simulink model "PowerTrainModeling"  (R2016a)
settings: Solver=ode3  StartTime=0.0  StopTime=1220  FixedStep=0.1  RelTol=1e-3
libraries: simulink x6
(part 3 of 3)

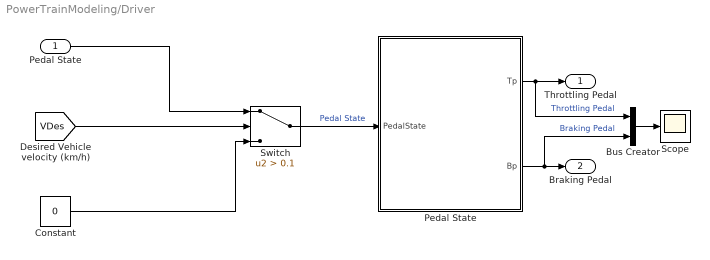
== system PowerTrainModeling/Driver ==
  "Pedal State " : Inport
  Bus Creator : BusCreator  Inputs=2
  Constant : Constant  Value=0
  Pedal State : MATLAB Function  TreatAsAtomicUnit=on
  Scope : Scope
  Switch : Switch  Criteria=u2 > Threshold  Threshold=0.1
  Throttling Pedal : Outport
  Braking Pedal : Outport  Port=2
  wires:
  Pedal State/2(Bp) -> Bus Creator/2, Braking Pedal/1  "Braking Pedal"
  Switch/1 -> Pedal State/1(PedalState)  "Pedal State"
  Constant/1 -> Switch/3
  [VDes] -> Switch/2
  Pedal State/1(Tp) -> Bus Creator/1, Throttling Pedal/1  "Throttling Pedal"
  "Pedal State "/1 -> Switch/1
  Bus Creator/1 -> Scope/1

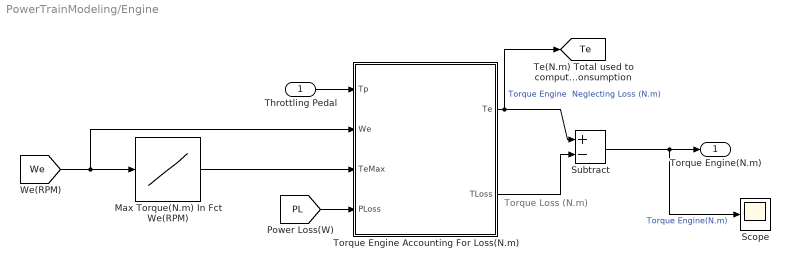
== system PowerTrainModeling/Engine  ==
  note: Torque Loss
      | (N.m)
  Throttling Pedal : Inport
  Max Torque(N.m) In Fct We(RPM) : Lookup_n-D  NumberOfTableDimensions=1  BreakpointsForDimension1=|  Table=|  RndMeth=Simplest  InputSameDT=on
      BreakpointsForDimension1=|
      | [500
      | 1000
      | 1500
      | 2000
      | 2500
      | 3000
      | 3500
      | 4000
      | 4500
      | 5000
      | 5500
      | 6000
      | ]
      Table=|
      | [112.32
      | 134.16
      | 146.64
      | 158.34
      | 165.36
      | 162.24
      | 159.12
      | 159.9
      | 165.36
      | 164.58
      | 160.68
      | 151.32
      | ]
  Scope : Scope
  Subtract : Sum  Inputs=+-
  Torque Engine Accounting For Loss(N.m) : MATLAB Function  TreatAsAtomicUnit=on
  Torque Engine(N.m) : Outport
  tag scope: Te=global
  wires:
  Max Torque(N.m) In Fct We(RPM)/1 -> Torque Engine Accounting For Loss(N.m)/3(TeMax)
  Torque Engine Accounting For Loss(N.m)/1(Te) -> [Te], Subtract/1  "Torque Engine  Neglecting Loss (N.m)"
  Subtract/1 -> Scope/1, Torque Engine(N.m)/1  "Torque Engine(N.m)"
  Throttling Pedal/1 -> Torque Engine Accounting For Loss(N.m)/1(Tp)
  [PL] -> Torque Engine Accounting For Loss(N.m)/4(PLoss)
  Torque Engine Accounting For Loss(N.m)/2(TLoss) -> Subtract/2
  [We] -> Torque Engine Accounting For Loss(N.m)/2(We), Max Torque(N.m) In Fct We(RPM)/1

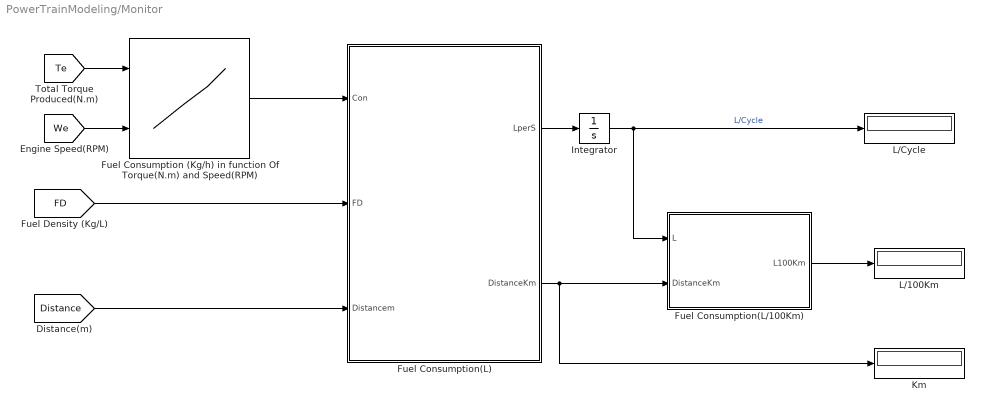
== system PowerTrainModeling/Monitor ==
  Fuel Consumption (Kg/h) in function Of Torque(N.m) and Speed(RPM) : Lookup_n-D  BreakpointsForDimension1=|  BreakpointsForDimension2=|  Table=|  RndMeth=Simplest  InputSameDT=on
      BreakpointsForDimension1=|
      | [15.6
      | 31.2
      | 46.8
      | 62.4
      | 78
      | 93.6
      | 109.2
      | 124.8
      | 140.4
      | 156
      | 171.6
      | ]
      Table=|
      | [0.50	1.00	1.50	1.94	2.28	2.56	2.68	3.41	3.97	5.59	6.79	7.41
      | 0.72	1.32	1.99	2.59	3.12	3.58	3.89	4.66	5.77	7.53	9.19	10.37
      | 0.91	1.65	2.54	3.28	3.93	4.58	4.94	6.22	7.75	9.26	11.35	12.70
      | 1.08	2.01	3.00	3.93	4.65	5.47	6.42	7.95	9.32	10.88	13.13	14.68
      | 1.25	2.32	3.44	4.50	5.44	6.44	7.92	9.23	10.78	12.50	14.72	16.41
      | 1.53	2.81	3.86	5.08	6.04	7.52	9.18	10.80	12.31	13.94	15.91	18.42
      | 1.73	3.23	4.37	5.60	7.00	8.52	10.37	12.02	13.99	16.20	18.79	20.50
      | 2.12	3.72	4.83	6.40	8.00	9.60	11.36	13.27	15.88	18.23	21.22	23.15
      | 2.12	4.23	5.56	7.30	9.00	10.80	12.78	15.46	18.05	20.80	23.58	25.72
      | 2.35	4.70	7.06	8.59	10.44	12.70	15.03	17.41	20.25	23.23	26.04	28.23
      | 2.59	5.18	7.76	10.35	12.94	15.53	18.11	20.70	23.29	25.88	28.46	31.05
      | ]
      BreakpointsForDimension2=|
      | [500	1000	1500	2000	2500	3000	3500	4000	4500	5000	5500	6000
      | ]
  Fuel Consumption(L) : MATLAB Function  TreatAsAtomicUnit=on
  Fuel Consumption(L/100Km) : MATLAB Function  TreatAsAtomicUnit=on
  Integrator : Integrator
  Km : Display
  L/100Km : Display
  L/Cycle : Display
  wires:
  [We] -> Fuel Consumption (Kg/h) in function Of Torque(N.m) and Speed(RPM)/2
  [Te] -> Fuel Consumption (Kg/h) in function Of Torque(N.m) and Speed(RPM)/1
  Fuel Consumption(L)/1(LperS) -> Integrator/1
  [FD] -> Fuel Consumption(L)/2(FD)
  Integrator/1 -> Fuel Consumption(L/100Km)/1(L), L/Cycle/1  "L/Cycle"
  Fuel Consumption(L)/2(DistanceKm) -> Km/1, Fuel Consumption(L/100Km)/2(DistanceKm)
  Fuel Consumption(L/100Km)/1(L100Km) -> L/100Km/1
  Fuel Consumption (Kg/h) in function Of Torque(N.m) and Speed(RPM)/1 -> Fuel Consumption(L)/1(Con)
  [Distance] -> Fuel Consumption(L)/3(Distancem)

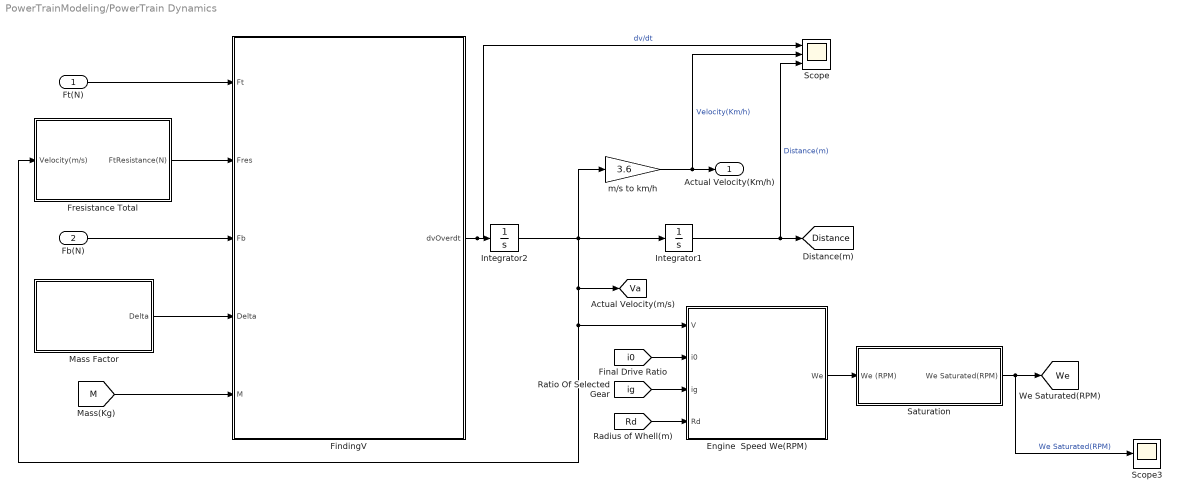
== system PowerTrainModeling/PowerTrain Dynamics  ==
  Ft(N) : Inport
  Fb(N) : Inport  Port=2
  Engine  Speed We(RPM) : MATLAB Function  TreatAsAtomicUnit=on
  FindingV : MATLAB Function  TreatAsAtomicUnit=on
  "Fresistance Total " : Subsystem
  Integrator1 : Integrator
  Integrator2 : Integrator
  Mass Factor : Subsystem
  Saturation : Subsystem
  Scope : Scope  NumInputPorts=3
  Scope3 : Scope
  m/s to km/h : Gain  Gain=3.6
  " Actual Velocity(Km/h)" : Outport
  tag scope: Distance=global, Va=global, We=global
  wires:
  "Fresistance Total "/1(FtResistance(N)) -> FindingV/2(Fres)
  Integrator1/1 -> Scope/3, [Distance]  "Distance(m)"
  FindingV/1(dvOverdt) -> Scope/1, Integrator2/1  "dv/dt"
  [M] -> FindingV/5(M)
  Ft(N)/1 -> FindingV/1(Ft)
  Mass Factor/1(Delta) -> FindingV/4(Delta)
  m/s to km/h/1 -> Scope/2, " Actual Velocity(Km/h)"/1  "Velocity(Km/h)"
  Fb(N)/1 -> FindingV/3(Fb)
  [ig] -> Engine  Speed We(RPM)/3(ig)
  [i0] -> Engine  Speed We(RPM)/2(i0)
  [Rd] -> Engine  Speed We(RPM)/4(Rd)
  Engine  Speed We(RPM)/1(We) -> Saturation/1(We (RPM))
  Saturation/1(We Saturated(RPM)) -> Scope3/1, [We]  "We Saturated(RPM)"
  Integrator2/1 -> m/s to km/h/1, Integrator1/1, "Fresistance Total "/1(Velocity(m/s)), Engine  Speed We(RPM)/1(V), [Va]

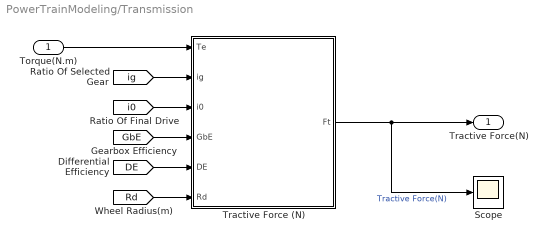
== system PowerTrainModeling/Transmission ==
  Torque(N.m) : Inport
  Scope : Scope
  Tractive Force (N) : MATLAB Function  TreatAsAtomicUnit=on
  Tractive Force(N) : Outport
  wires:
  [DE] -> Tractive Force (N)/5(DE)
  [i0] -> Tractive Force (N)/3(i0)
  [GbE] -> Tractive Force (N)/4(GbE)
  [Rd] -> Tractive Force (N)/6(Rd)
  [ig] -> Tractive Force (N)/2(ig)
  Torque(N.m)/1 -> Tractive Force (N)/1(Te)
  Tractive Force (N)/1(Ft) -> Scope/1, Tractive Force(N)/1  "Tractive Force(N)"

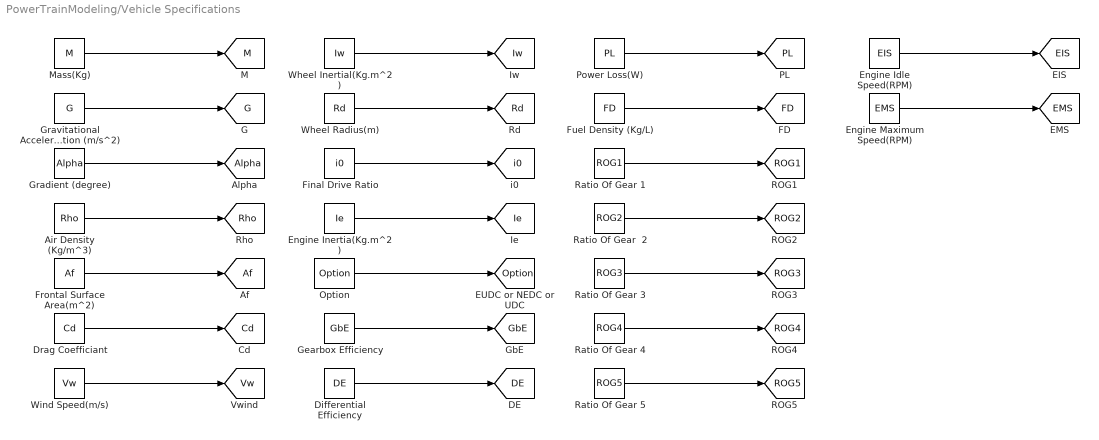
== system PowerTrainModeling/Vehicle Specifications ==
  Air Density (Kg/m^3) : Constant  Value=Rho
  Differential Efficiency : Constant  Value=DE
  Drag Coefficiant : Constant  Value=Cd
  Engine Idle Speed(RPM) : Constant  Value=EIS
  Engine Inertia(Kg.m^2) : Constant  Value=Ie
  Engine Maximum Speed(RPM) : Constant  Value=EMS
  Final Drive Ratio : Constant  Value=i0
  Frontal Surface Area(m^2) : Constant  Value=Af
  Fuel Density (Kg/L) : Constant  Value=FD
  Gearbox Efficiency : Constant  Value=GbE
  Gradient (degree) : Constant  Value=Alpha
  Gravitational Acceleration (m/s^2) : Constant  Value=G
  Mass(Kg) : Constant  Value=M
  Option : Constant  Value=Option
  Power Loss(W) : Constant  Value=PL
  Ratio Of Gear  2 : Constant  Value=ROG2
  Ratio Of Gear 1 : Constant  Value=ROG1
  Ratio Of Gear 3 : Constant  Value=ROG3
  Ratio Of Gear 4 : Constant  Value=ROG4
  Ratio Of Gear 5 : Constant  Value=ROG5
  Wheel Inertial(Kg.m^2) : Constant  Value=Iw
  Wheel Radius(m) : Constant  Value=Rd
  Wind Speed(m/s) : Constant  Value=Vw
  tag scope: Af=global, Alpha=global, Cd=global, DE=global, EIS=global, EMS=global, FD=global, G=global, GbE=global, Ie=global, Iw=global, M=global, Option=global, PL=global, ROG1=global, ROG2=global, ROG3=global, ROG4=global, ROG5=global, Rd=global, Rho=global, Vw=global, i0=global
  wires:
  Engine Inertia(Kg.m^2)/1 -> [Ie]
  Final Drive Ratio/1 -> [i0]
  Wheel Radius(m)/1 -> [Rd]
  Wind Speed(m/s)/1 -> [Vw]
  Drag Coefficiant/1 -> [Cd]
  Frontal Surface Area(m^2)/1 -> [Af]
  Air Density (Kg/m^3)/1 -> [Rho]
  Gradient (degree)/1 -> [Alpha]
  Gravitational Acceleration (m/s^2)/1 -> [G]
  Mass(Kg)/1 -> [M]
  Option/1 -> [Option]
  Gearbox Efficiency/1 -> [GbE]
  Differential Efficiency/1 -> [DE]
  Power Loss(W)/1 -> [PL]
  Fuel Density (Kg/L)/1 -> [FD]
  Ratio Of Gear 1/1 -> [ROG1]
  Ratio Of Gear  2/1 -> [ROG2]
  Ratio Of Gear 5/1 -> [ROG5]
  Ratio Of Gear 4/1 -> [ROG4]
  Ratio Of Gear 3/1 -> [ROG3]
  Engine Idle Speed(RPM)/1 -> [EIS]
  Engine Maximum Speed(RPM)/1 -> [EMS]
  Wheel Inertial(Kg.m^2)/1 -> [Iw]

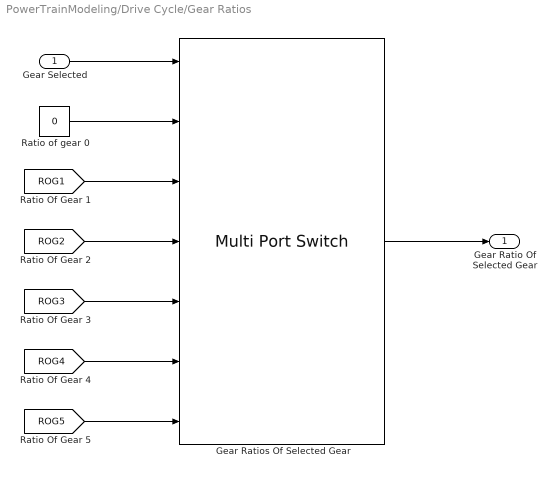
== system PowerTrainModeling/Drive Cycle/Gear Ratios  ==
  Gear Selected : Inport
  Gear Ratios Of Selected Gear : MultiPortSwitch  DataPortOrder=Specify indices  Inputs=6  DataPortIndices={0,1,2,3,4,5}
  Ratio of gear 0 : Constant  Value=0
  Gear Ratio Of Selected Gear : Outport
  wires:
  Gear Ratios Of Selected Gear/1 -> Gear Ratio Of Selected Gear/1
  Ratio of gear 0/1 -> Gear Ratios Of Selected Gear/2
  [ROG3] -> Gear Ratios Of Selected Gear/5
  [ROG4] -> Gear Ratios Of Selected Gear/6
  [ROG1] -> Gear Ratios Of Selected Gear/3
  [ROG2] -> Gear Ratios Of Selected Gear/4
  Gear Selected/1 -> Gear Ratios Of Selected Gear/1
  [ROG5] -> Gear Ratios Of Selected Gear/7

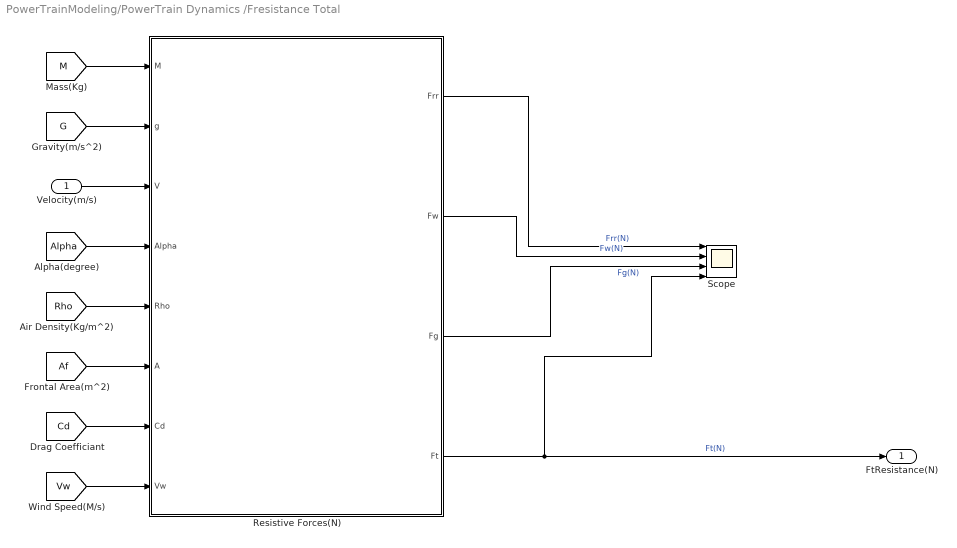
== system PowerTrainModeling/PowerTrain Dynamics /Fresistance Total  ==
  Velocity(m/s) : Inport
  " Resistive Forces(N)" : MATLAB Function  TreatAsAtomicUnit=on
  Scope : Scope  NumInputPorts=4
  FtResistance(N) : Outport
  wires:
  Velocity(m/s)/1 -> " Resistive Forces(N)"/3(V)
  " Resistive Forces(N)"/4(Ft) -> Scope/4, FtResistance(N)/1  "Ft(N)"
  [Rho] -> " Resistive Forces(N)"/5(Rho)
  " Resistive Forces(N)"/2(Fw) -> Scope/2  "Fw(N)"
  " Resistive Forces(N)"/1(Frr) -> Scope/1  "Frr(N)"
  [Vw] -> " Resistive Forces(N)"/8(Vw)
  [Cd] -> " Resistive Forces(N)"/7(Cd)
  [Af] -> " Resistive Forces(N)"/6(A)
  [Alpha] -> " Resistive Forces(N)"/4(Alpha)
  [G] -> " Resistive Forces(N)"/2(g)
  [M] -> " Resistive Forces(N)"/1(M)
  " Resistive Forces(N)"/3(Fg) -> Scope/3  "Fg(N)"

== system PowerTrainModeling/PowerTrain Dynamics /Mass Factor ==
  Mass Factor : MATLAB Function  TreatAsAtomicUnit=on
  Scope : Scope
  Delta : Outport
  wires:
  [i0] -> Mass Factor/4(i0)
  [Ie] -> Mass Factor/6(Ie)
  [M] -> Mass Factor/2(M)
  [Iw] -> Mass Factor/1(Iw)
  Mass Factor/1(MassFactor) -> Scope/1, Delta/1  "Delta"
  [Rd] -> Mass Factor/3(Rd)
  [ig] -> Mass Factor/5(ig)

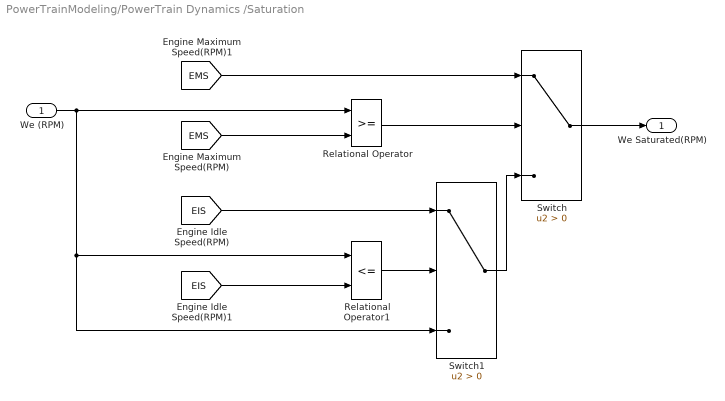
== system PowerTrainModeling/PowerTrain Dynamics /Saturation ==
  We (RPM) : Inport
  Relational Operator : RelationalOperator  OutDataTypeStr=boolean
  Relational Operator1 : RelationalOperator  Operator=<=  OutDataTypeStr=boolean
  Switch : Switch  Criteria=u2 > Threshold
  Switch1 : Switch  Criteria=u2 > Threshold
  We Saturated(RPM) : Outport
  wires:
  [EMS] -> Switch/1
  Relational Operator/1 -> Switch/2
  Switch/1 -> We Saturated(RPM)/1
  [EMS] -> Relational Operator/2
  Relational Operator1/1 -> Switch1/2
  Switch1/1 -> Switch/3
  [EIS] -> Switch1/1
  We (RPM)/1 -> Relational Operator1/1, Switch1/3, Relational Operator/1
  [EIS] -> Relational Operator1/2

== matlab function PowerTrainModeling/PowerTrain Dynamics /Mass Factor/Mass Factor ==
  data: Iw input; MassFactor output; M input; Rd input; i0 input; ig input; Ie input


function MassFactor =Delta(Iw,M,Rd,i0,ig,Ie)
%1st component
first=1;
%2nd component
second=Iw/(M*(Rd^2));
%3rd component
third=((i0^2)*(ig^2)*Ie)/(M*(Rd^2));
MassFactor=first+second+third;

== matlab function PowerTrainModeling/PowerTrain Dynamics /Fresistance Total / Resistive Forces(N) ==
  data: Frr output; M input; Fw output; g input; Fg output; V input; Alpha input; Rho input; A input; Cd input; Vw input; Ft output


function [Frr,Fw,Fg,Ft]=Ftresistance(M,g,V,Alpha,Rho,A,Cd,Vw)


% frr
frr=0.01+(0.00036*V);
% Force rollig Resistance (N)
Frr=M*g*frr*cos(Alpha);
%Force Wind(N)
Fw=0.5*Rho*A*Cd*((V+Vw)^2);
%Force Gradient(N)
Fg=M*g*sin(Alpha);

%condition for negative Velocity or Velocity equal 0%if(V>0)
%Total Resistive Forces(N)
if(V>0)
Ft=Frr+Fw+Fg;
else
    Ft=0;
end

== matlab function PowerTrainModeling/PowerTrain Dynamics /FindingV ==
  data: dvOverdt output; Ft input; Fres input; Fb input; Delta input; M input


function dvOverdt =FindingV(Ft,Fres,Fb,Delta,M)
dvOverdt =(Ft-Fres-Fb)/(Delta*M);

== matlab function PowerTrainModeling/PowerTrain Dynamics /Engine  Speed We(RPM) ==
  data: We output; V input; i0 input; ig input; Rd input


function We =We(V,i0,ig,Rd)
We=(V*30*ig*i0)/(pi*Rd);
end

== matlab function PowerTrainModeling/Transmission/Tractive Force (N) ==
  data: Ft output; Te input; ig input; i0 input; GbE input; DE input; Rd input


function Ft =TractiveForce(Te,ig,i0,GbE,DE,Rd)
Ft=(Te*ig*i0*GbE*DE)/Rd;




end

== matlab function PowerTrainModeling/Engine /Torque Engine Accounting For Loss(N.m) ==
  data: Tp input; We input; Te output; TeMax input; TLoss output; PLoss input


function [Te,TLoss] =Torque(Tp,We,TeMax,PLoss)
% Neglecting Loss and Finding Engine Torque (N.m)
Te=Tp*TeMax;
% Torque Loss(N.m)
if(Tp>0)
TLoss=(30*PLoss)/(pi*We);
else
    TLoss=0;
end

== matlab function PowerTrainModeling/Monitor/Fuel Consumption(L) ==
  data: LperS output; Con input; FD input; Distancem input; DistanceKm output


function [LperS,DistanceKm]  =FuelConsumption(Con,FD,Distancem)
% Fuel consumption in L per s Dividing by Fuel density and conversion h to s
LperS=Con/(FD*3600);
% Convert from distance in m to Km
DistanceKm=Distancem*0.001;


end

== matlab function PowerTrainModeling/Monitor/Fuel Consumption(L//100Km) ==
  data: L input; L100Km output; DistanceKm input


function L100Km =FC(L,DistanceKm)
% Consumption in Litre per 100 Km


L100Km=(L*100)/DistanceKm;

       

end

== matlab function PowerTrainModeling/Driver/Pedal State ==
  data: Tp output; PedalState input; Bp output


function [Tp,Bp] =Pedal(PedalState)
if(PedalState>0)
Tp=PedalState;
else
Tp=0;
end

if(PedalState<0)
Bp=abs(PedalState);
else
Bp=0;
end
